simulink model "QuadcopterControlInput"  (R2023b)
settings: Solver=VariableStepAuto  StartTime=0.0  StopTime=10.0  RelTol=1e-3
values from neighbouring files (symbols this model uses):
  Kf = 3.13e-5    (= 3.13e-05)    [QuadcopterParameters.m]
  Km = 7.5e-7    (= 7.5e-07)    [QuadcopterParameters.m]
undefined symbols (not defined in the file or in its folder): magnitude

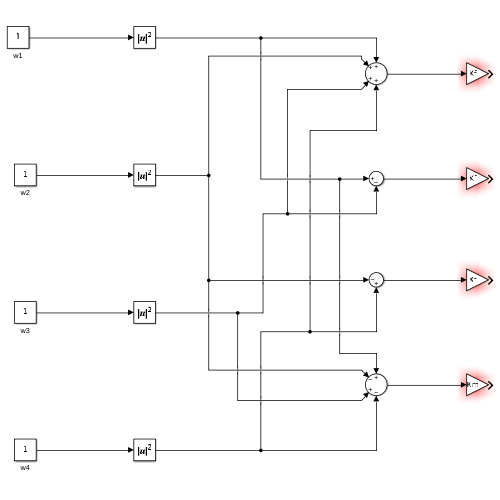
[thumbnail: Simulink's stored preview of the top-level diagram]
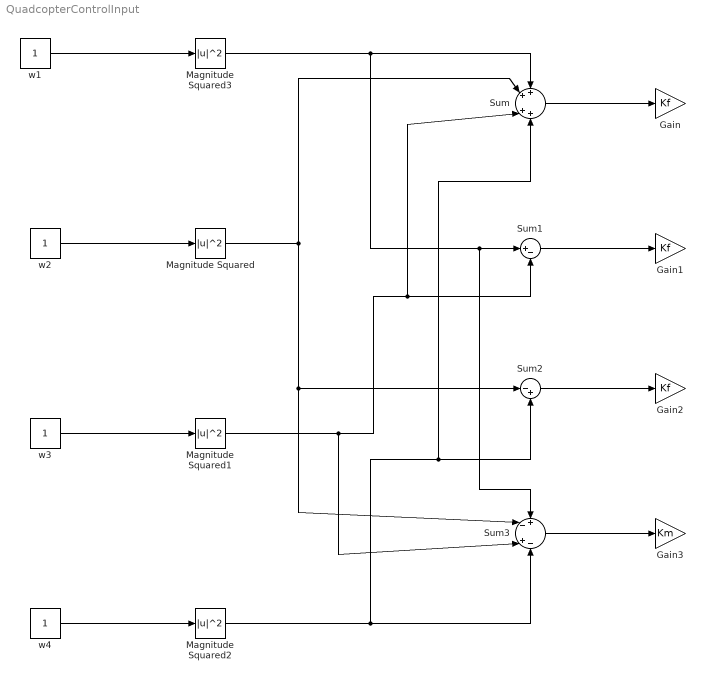
== system QuadcopterControlInput ==
  Gain : Gain  Gain=Kf
  Gain1 : Gain  Gain=Kf
  Gain2 : Gain  Gain=Kf
  Gain3 : Gain  Gain=Km
  Magnitude Squared{,1..3} (4 alike) : Math  Operator=magnitude^2
  Sum : Sum  Inputs=++|++
  Sum1 : Sum  Inputs=|+-
  Sum2 : Sum  Inputs=|-+
  Sum3 : Sum  Inputs=+-|+-
  w{1..4} (4 alike) : Constant
  wires:
  Magnitude Squared3/1 -> Sum/1, Sum3/1, Sum1/1
  Magnitude Squared1/1 -> Sum3/3, Sum/3, Sum1/2
  Magnitude Squared/1 -> Sum/2, Sum2/1, Sum3/2
  Magnitude Squared2/1 -> Sum3/4, Sum2/2, Sum/4
  Sum1/1 -> Gain1/1
  Sum/1 -> Gain/1
  Sum2/1 -> Gain2/1
  Sum3/1 -> Gain3/1
  w1/1 -> Magnitude Squared3/1
  w3/1 -> Magnitude Squared1/1
  w4/1 -> Magnitude Squared2/1
  w2/1 -> Magnitude Squared/1
